simulink model "fz5_16"  (R2014a)
settings: Solver=ode45  StartTime=0.0  StopTime=10.0  MaxStep=0.001  RelTol=1e-3
undefined symbols (not defined in the file or in its folder): magnitude
libraries: dspstat3 x2, commanapbnd3 x1, commrandsrc2 x1
settings Model: Creator=tzb  LastModifiedBy=tzb

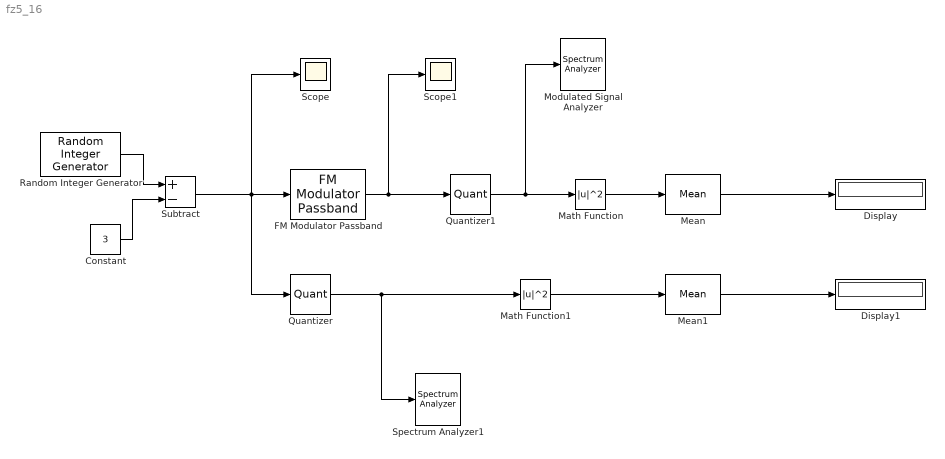
== system fz5_16 ==
  Constant : Constant  Value=3
  Display : Display
  Display1 : Display
  FM Modulator Passband : commanapbnd3/FM Modulator Passband  Fc=250  Ph=0  Kc=50
  Math Function : Math  Operator=magnitude^2  SaturateOnIntegerOverflow=on
  Math Function1 : Math  Operator=magnitude^2  SaturateOnIntegerOverflow=on
  Mean : dspstat3/Mean  run=on  reset_popup=None  InputProcessing=Columns as channels (frame based)  directionMode=Each column  dimension=1  treatSBRowAsCol=on  roiEnable=off  roiType=Rectangles  roiPortion=Entire ROI  roiOutput=Individual statistics for each ROI  roiFlag=off  outputDataTypeStr=Inherit: Same as accumulator  outputLastDataTypeStr=Inherit: Same as accumulator  outputMin=[]  outputMax=[]  roundingMode=Floor  overflowMode=off
  Mean1 : dspstat3/Mean  run=on  reset_popup=None  InputProcessing=Columns as channels (frame based)  directionMode=Each column  dimension=1  treatSBRowAsCol=on  roiEnable=off  roiType=Rectangles  roiPortion=Entire ROI  roiOutput=Individual statistics for each ROI  roiFlag=off  outputDataTypeStr=Inherit: Same as accumulator  outputLastDataTypeStr=Inherit: Same as accumulator  outputMin=[]  outputMax=[]  roundingMode=Floor  overflowMode=off
  Modulated Signal Analyzer : SpectrumAnalyzer
  Quantizer : Quantizer  QuantizationInterval=0.001  LinearizeAsGain=off  SampleTime=0.001
  Quantizer1 : Quantizer  QuantizationInterval=0.001  LinearizeAsGain=off  SampleTime=0.001
  Random Integer Generator : commrandsrc2/Random Integer Generator  mul=7  seed=37  Ts=1/10  frameBased=off  sampPerFrame=1  orient=off  outDataType=double
  Scope : Scope
  Scope1 : Scope
  Spectrum Analyzer1 : SpectrumAnalyzer
  Subtract : Sum  Inputs=+-
  wires:
  Random Integer Generator/1 -> Subtract/1
  Constant/1 -> Subtract/2
  Math Function/1 -> Mean/1
  Mean/1 -> Display/1
  Subtract/1 -> Quantizer/1, Scope/1, FM Modulator Passband/1
  FM Modulator Passband/1 -> Quantizer1/1, Scope1/1
  Quantizer1/1 -> Modulated Signal Analyzer/1, Math Function/1
  Quantizer/1 -> Spectrum Analyzer1/1, Math Function1/1
  Math Function1/1 -> Mean1/1
  Mean1/1 -> Display1/1
